simulink model "ev_phase3"  (R2025a)
settings: Solver=VariableStepAuto  StartTime=0.0  StopTime=3600  RelTol=1e-3
libraries: SignalEditorBlockLib x2
settings Model: Creator=piyus  LastModifiedBy=piyus

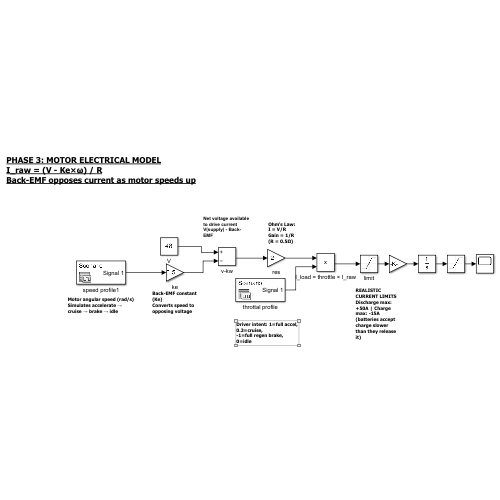
[thumbnail: Simulink's stored preview of the top-level diagram]
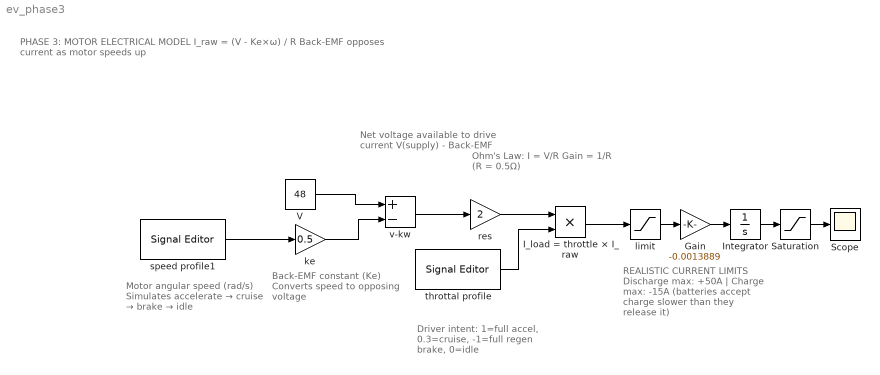
== system ev_phase3 ==
  note: REALISTIC CURRENT LIMITS
      | Discharge max: +50A | Charge max: -15A
      | (batteries accept charge slower than they release it)
  note: Driver intent: 1=full accel, 0.3=cruise,
      | -1=full regen brake, 0=idle
  note: Ohm's Law: I = V/R
      | Gain = 1/R (R = 0.5Ω)
  note: Net voltage available to drive current
      | V(supply) - Back-EMF
  note: Back-EMF constant (Ke)
      | Converts speed to opposing voltage
  note: Motor angular speed (rad/s)
      | Simulates accelerate → cruise → brake → idle
  note: PHASE 3: MOTOR ELECTRICAL MODEL
      | I_raw = (V - Ke×ω) / R
      | Back-EMF opposes current as motor speeds up
  Gain : Gain  Gain=-0.0013889
  I_load = throttle × I_raw : Product
  Integrator : Integrator  InitialCondition=100
  Saturation : Saturate  UpperLimit=100  LowerLimit=0
  Scope : Scope
      settings: ActiveDisplayYMinimum=-135.8301484940319  ActiveDisplayYMaximum=199.19376166221778
  V : Constant  Value=48
  ke : Gain  Gain=0.5
  limit : Saturate  UpperLimit=50  LowerLimit=-15
  res : Gain  Gain=2
  speed profile1 : SignalEditorBlockLib/Signal Editor  FileName=speed_profile.mat  ActiveScenario=Scenario  ActiveSignal=Signal 1  IsBus=off  OutputBusObjectStr=Bus: BusObject  SampleTime=0  ZeroCross=off  OutputAfterFinalValue=Setting to zero  Unit=inherit  PreserveSignalName=on  ApplySigPropsToAllScenarios=on  ApplySigPropsToAllSignals=off  SignalPropertySource=Dialog parameters
  throttal profile : SignalEditorBlockLib/Signal Editor  FileName=throttle_profile.mat  ActiveScenario=Scenario  ActiveSignal=Signal 1  IsBus=off  OutputBusObjectStr=Bus: BusObject  SampleTime=0  ZeroCross=off  OutputAfterFinalValue=Setting to zero  Unit=inherit  PreserveSignalName=on  ApplySigPropsToAllScenarios=on  ApplySigPropsToAllSignals=off  SignalPropertySource=Dialog parameters
  v-kw : Sum  Inputs=+-
  wires:
  speed profile1/1 -> ke/1
  V/1 -> v-kw/1
  ke/1 -> v-kw/2
  v-kw/1 -> res/1
  res/1 -> I_load = throttle × I_raw/1
  throttal profile/1 -> I_load = throttle × I_raw/2
  Integrator/1 -> Saturation/1
  Saturation/1 -> Scope/1
  Gain/1 -> Integrator/1
  I_load = throttle × I_raw/1 -> limit/1
  limit/1 -> Gain/1
